simulink model "mimoSimulation_noInit_uncertain"  (R2013b)
settings: Solver=ode45  StartTime=0.0  StopTime=0.3  RelTol=1e-5
values from neighbouring files (symbols this model uses):
  act = ss( rsys )    [evalDMSim_uncertain.m]
  delay = Ts*2    (= 0.00117647058824)    [evalDMSim_uncertain.m]
  K1_disk = c2d(K1, Ts)    [evalDMSim_uncertain.m]
  sizeDM = 24    [evalDMSim_uncertain.m]
  Ts = 1/1700    (= 0.000588235294118)    [evalDMSim_uncertain.m]
undefined symbols (not defined in the file or in its folder): ultidyn
libraries: simulink x1, RCTblocks x1
settings Model: Creator=steffen  LastModifiedBy=smauch
settings DataIOCC: SignalLoggingSaveFormat=ModelDataLogs
settings OptimizationCC: ExpressionDepthLimit=2147483647  SimCompilerOptimization=On
settings DebuggingCC: FcnCallInpInsideContextMsg=UseLocalSettings  StateNameClashWarn=warning
settings GRTTargetCC: CombineOutputUpdateFcns=off  GRTInterface=on

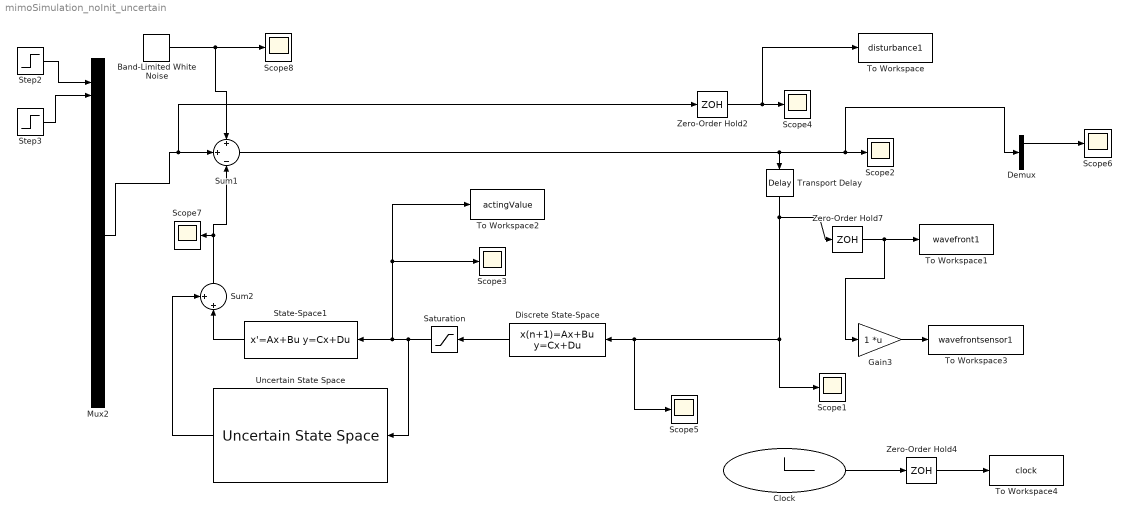
== system mimoSimulation_noInit_uncertain ==
  Band-Limited White Noise : simulink/Sources/Band-Limited White Noise  Cov=diag(sizeDM)*0.0002*0.0005*0.05  Ts=0.005  seed=round(abs(randn(sizeDM,1))*1000)
  Clock : Clock
  Demux : Demux  Outputs=[1 23]
  Discrete State-Space : DiscreteStateSpace  A=K1_disk.A  B=K1_disk.B  C=K1_disk.C  D=K1_disk.D  SampleTime=Ts
  Gain3 : Gain  Multiplication=Matrix(K*u)
  Mux2 : Mux  Inputs=sizeDM
  Saturation : Saturate  UpperLimit=1  LowerLimit=-1
  Scope{1..8} (8 alike) : Scope
      Scope1 settings: TimeRange=0.6  YMin=0.55  YMax=1.025
      Scope2 settings: TimeRange=0.8  YMin=0.008890127388535037  YMax=0.02689012738853504  SaveName=ScopeData2
      Scope3 settings: TimeRange=0.08631415241057544  YMin=-0.08666666666666628  YMax=1.372
      Scope4 settings: TimeRange=2  YMin=-0.1  YMax=0.8  SaveName=ScopeData3
      Scope5 settings: TimeRange=0.6  YMin=0.55  YMax=1.025  SaveName=ScopeData4
      Scope6 settings: TimeRange=0.8  YMin=0.0383  YMax=0.0398  SaveName=ScopeData5
      Scope7 settings: TimeRange=0.7000000000000001  YMin=0  YMax=10  SaveName=ScopeData7
      Scope8 settings: TimeRange=0.8  YMin=0.0383  YMax=0.0398  SaveName=ScopeData6
  State-Space1 : StateSpace  A=act.A  B=act.B  C=act.C  D=act.D  X0=0
  Step2 : Step  Time=0.15  After=-0.1  SampleTime=0
  Step3 : Step  Time=0.1  After=-0.2  SampleTime=0
  Sum1 : Sum  Inputs=+|+|-
  Sum2 : Sum  Inputs=+|+||
  To Workspace : ToWorkspace  VariableName=disturbance1  SampleTime=-1  SaveFormat=Structure
  To Workspace1 : ToWorkspace  VariableName=wavefront1  SampleTime=-1  SaveFormat=Structure
  To Workspace2 : ToWorkspace  VariableName=actingValue  SampleTime=-1  SaveFormat=Structure
  To Workspace3 : ToWorkspace  VariableName=wavefrontsensor1  SampleTime=-1  SaveFormat=Structure
  To Workspace4 : ToWorkspace  VariableName=clock  SampleTime=-1  SaveFormat=Structure
  Transport Delay : TransportDelay  DelayTime=delay  BufferSize=4096
  Uncertain State Space : RCTblocks/Uncertain State Space  Tag=USS  USystem=ultidyn( 'deltaDM',[sizeDM sizeDM],'Bound',1)/20  UValue=uval  X0=[]  uX0=[]
  Zero-Order Hold2 : ZeroOrderHold  SampleTime=Ts
  Zero-Order Hold4 : ZeroOrderHold  SampleTime=Ts
  Zero-Order Hold7 : ZeroOrderHold  SampleTime=Ts
  wires:
  Mux2/1 -> Sum1/2, Zero-Order Hold2/1
  Discrete State-Space/1 -> Saturation/1
  Clock/1 -> Zero-Order Hold4/1
  Zero-Order Hold4/1 -> To Workspace4/1
  Zero-Order Hold7/1 -> To Workspace1/1, Gain3/1
  Band-Limited White Noise/1 -> Sum1/1, Scope8/1
  Zero-Order Hold2/1 -> Scope4/1, To Workspace/1
  Step3/1 -> Mux2/2
  Step2/1 -> Mux2/1
  Gain3/1 -> To Workspace3/1
  Sum1/1 -> Transport Delay/1, Demux/1, Scope2/1
  Demux/1 -> Scope6/1
  Saturation/1 -> Uncertain State Space/1, State-Space1/1, To Workspace2/1, Scope3/1
  State-Space1/1 -> Sum2/2
  Sum2/1 -> Scope7/1, Sum1/3
  Uncertain State Space/1 -> Sum2/1
  Transport Delay/1 -> Scope5/1, Discrete State-Space/1, Scope1/1, Zero-Order Hold7/1
